simulink model "Speed_c_code_Testing_Pract"  (R2022a)
settings: Solver=VariableStepAuto  StartTime=0.0  StopTime=10  RelTol=1e-3
undefined symbols (not defined in the file or in its folder): d, F_0, F_0k, g, m, M, P_0, P_0k, PD_s, PI_s, Ts, V_0, V_0k
settings Model: Creator=DELL  LastModifiedBy=DELL

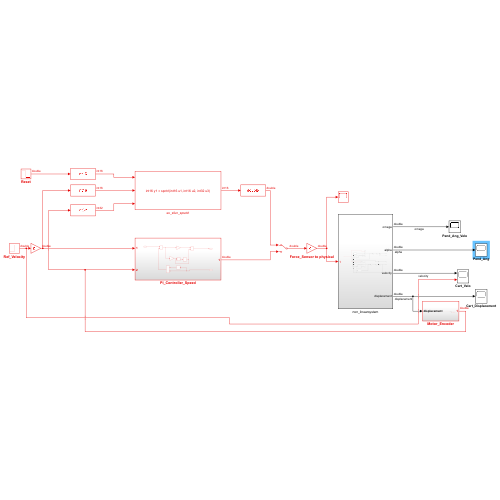
[thumbnail: Simulink's stored preview of the top-level diagram]
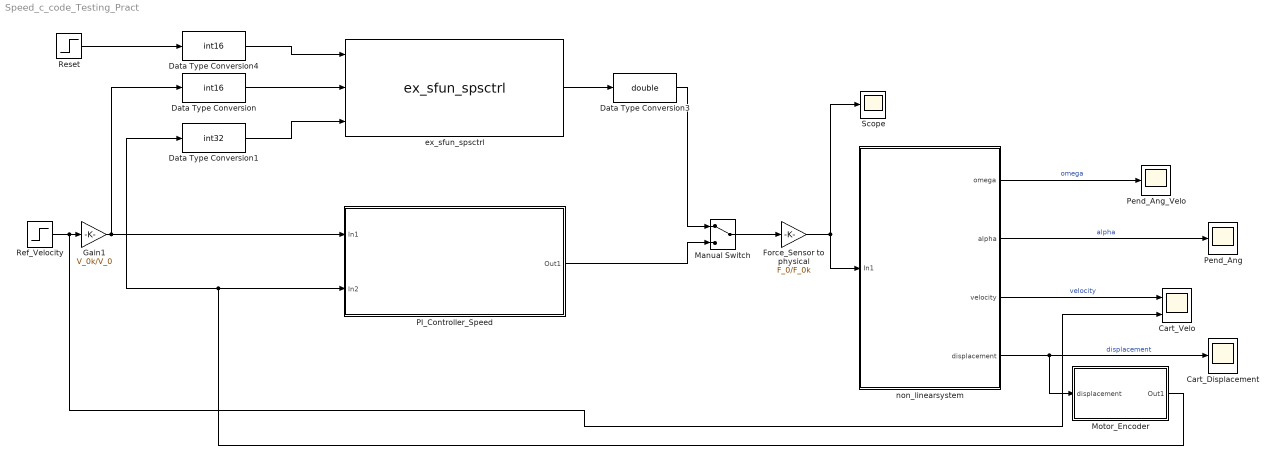
== system Speed_c_code_Testing_Pract ==
  Cart_Displacement : Scope
  Cart_Velo : Scope  NumInputPorts=2
  Data Type Conversion : DataTypeConversion  OutDataTypeStr=int16  SaturateOnIntegerOverflow=off  RndMeth=Floor
  Data Type Conversion1 : DataTypeConversion  OutDataTypeStr=int32  SaturateOnIntegerOverflow=off  RndMeth=Floor
  Data Type Conversion3 : DataTypeConversion  OutDataTypeStr=double  SaturateOnIntegerOverflow=off  RndMeth=Floor
  Data Type Conversion4 : DataTypeConversion  OutDataTypeStr=int16  SaturateOnIntegerOverflow=off  RndMeth=Floor
  Force_Sensor to physical : Gain  Gain=F_0/F_0k
  Gain1 : Gain  Gain=V_0k/V_0
  Manual Switch : ManualSwitch
  Motor_Encoder : Subsystem
  PI_Controller_Speed : Subsystem
  Pend_Ang : Scope
  Pend_Ang_Velo : Scope
  Ref_Velocity : Step  SampleTime=Ts
  Reset : Step  Time=2*Ts  Before=1  After=0  SampleTime=Ts
  Scope : Scope
  ex_sfun_spsctrl : S-Function  FunctionName=ex_sfun_spsctrl  SFunctionDeploymentMode=off  EnableBusSupport=off  mask(Legacy Function){SFunctionSpec=int16 y1 = spctrl(int16 u1, int16 u2, int32 u3), ShowSpec=on}
      mask prompts: ShowSpec "Display function specification"
      mask help:
      | This block allows you to call the legacy functions specified by the following Legacy Code Tool definition:
      | def.SFunctionName = 'ex_sfun_spsctrl';
      | def.OutputFcnSpec = 'int16 y1 = spctrl(int16 u1, int16 u2, int32 u3)';
      | def.HeaderFiles = {'xil_types.h', 'Fixedpt_Speed_Control.h'};
      mask Help: <p>This block was generated automatically by the Legacy Code Tool. For detailed help on this tool, call<a href="matlab:legacy_code('help')"> legacy_code('help')</a>.</p>
      mask Callback ShowSpec:
      | if strcmp(get_param(gcbh, 'ShowSpec'), 'on')
      |   set_param(gcbh, 'MaskDisplay', sprintf('fprintf(''%s'');', get_param(gcbh, 'SFunctionSpec')));
      | else
      |   set_param(gcbh, 'MaskDisplay', sprintf('fprintf(''%s'');', get_param(gcbh, 'FunctionName')));
      | end
      mask Display: fprintf('int16 y1 = spctrl(int16 u1, int16 u2, int32 u3)');
  non_linearsystem : Subsystem
  wires:
  non_linearsystem/1(omega) -> Pend_Ang_Velo/1  "omega"
  non_linearsystem/2(alpha) -> Pend_Ang/1  "alpha"
  non_linearsystem/3(velocity) -> Cart_Velo/1  "velocity"
  non_linearsystem/4(displacement) -> Motor_Encoder/1(displacement), Cart_Displacement/1  "displacement"
  Data Type Conversion1/1 -> ex_sfun_spsctrl/3
  ex_sfun_spsctrl/1 -> Data Type Conversion3/1
  Data Type Conversion3/1 -> Manual Switch/1
  Manual Switch/1 -> Force_Sensor to physical/1
  Data Type Conversion/1 -> ex_sfun_spsctrl/2
  Reset/1 -> Data Type Conversion4/1
  Data Type Conversion4/1 -> ex_sfun_spsctrl/1
  Force_Sensor to physical/1 -> non_linearsystem/1(In1), Scope/1
  PI_Controller_Speed/1(Out1) -> Manual Switch/2
  Ref_Velocity/1 -> Cart_Velo/2, Gain1/1
  Motor_Encoder/1(Out1) -> Data Type Conversion1/1, PI_Controller_Speed/2(In2)
  Gain1/1 -> Data Type Conversion/1, PI_Controller_Speed/1(In1)

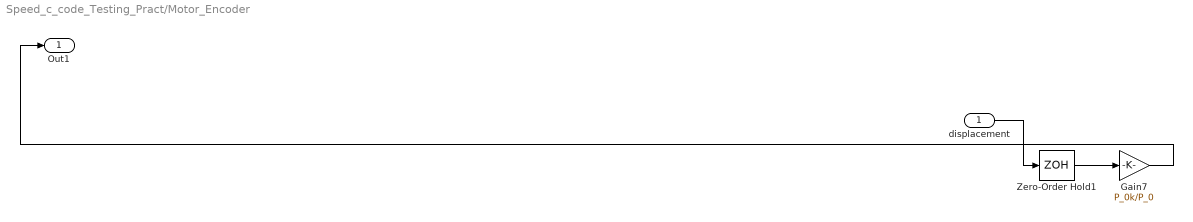
== system Speed_c_code_Testing_Pract/Motor_Encoder ==
  displacement : Inport
  Gain7 : Gain  Gain=P_0k/P_0
  Zero-Order Hold1 : ZeroOrderHold  SampleTime=Ts
  Out1 : Outport
  wires:
  Zero-Order Hold1/1 -> Gain7/1
  Gain7/1 -> Out1/1
  displacement/1 -> Zero-Order Hold1/1

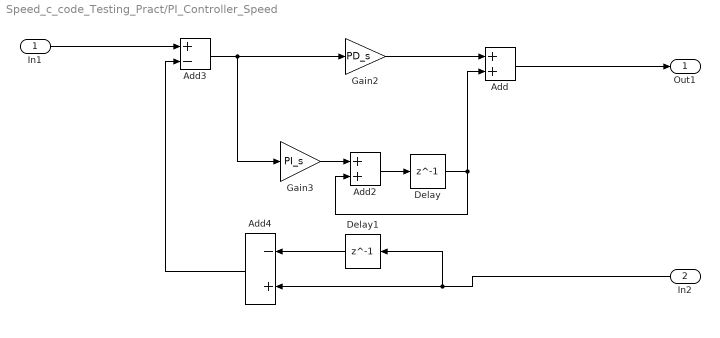
== system Speed_c_code_Testing_Pract/PI_Controller_Speed ==
  In1 : Inport
  In2 : Inport  Port=2
  Add : Sum
  Add2 : Sum
  Add3 : Sum  Inputs=+-
  Add4 : Sum  Inputs=-+
  Delay : Delay  DelayLength=1  SampleTime=Ts
  Delay1 : Delay  DelayLength=1  InitialCondition=0  SampleTime=Ts
  Gain2 : Gain  Gain=PD_s
  Gain3 : Gain  Gain=PI_s
  Out1 : Outport
  wires:
  Add/1 -> Out1/1
  Add3/1 -> Gain3/1, Gain2/1
  Gain2/1 -> Add/1
  Delay1/1 -> Add4/1
  Delay/1 -> Add/2, Add2/2
  In2/1 -> Add4/2, Delay1/1
  Add4/1 -> Add3/2
  Gain3/1 -> Add2/1
  Add2/1 -> Delay/1
  In1/1 -> Add3/1

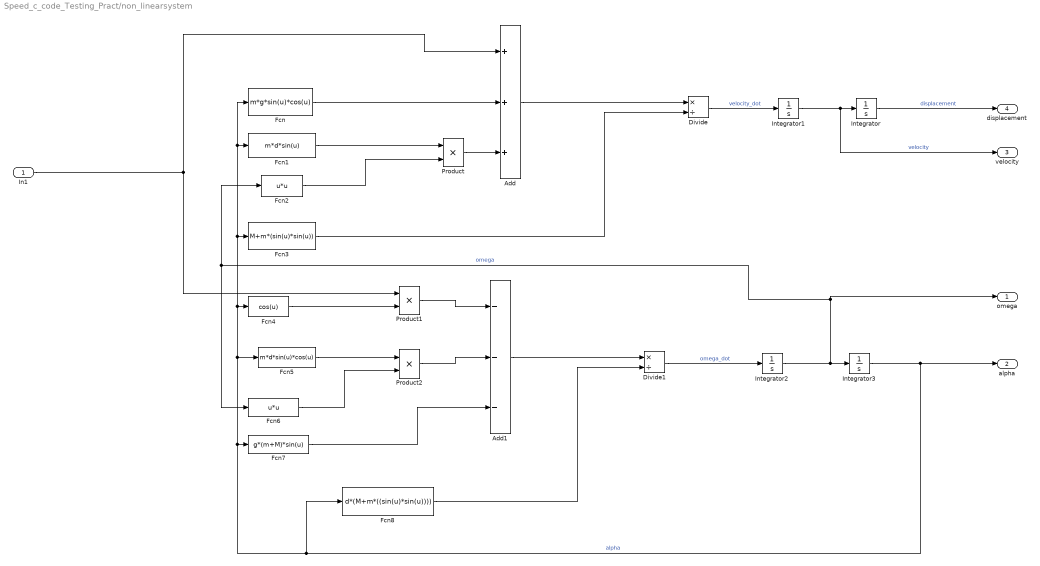
== system Speed_c_code_Testing_Pract/non_linearsystem ==
  In1 : Inport
  Add : Sum  Inputs=+++
  Add1 : Sum  Inputs=---
  Divide : Product  Inputs=*/
  Divide1 : Product  Inputs=*/
  Fcn : Fcn  Expr=m*g*sin(u)*cos(u)
  Fcn1 : Fcn  Expr=m*d*sin(u)
  Fcn2 : Fcn  Expr=u*u
  Fcn3 : Fcn  Expr=M+m*(sin(u)*sin(u))
  Fcn4 : Fcn  Expr=cos(u)
  Fcn5 : Fcn  Expr=m*d*sin(u)*cos(u)
  Fcn6 : Fcn  Expr=u*u
  Fcn7 : Fcn  Expr=g*(m+M)*sin(u)
  Fcn8 : Fcn  Expr=d*(M+m*((sin(u)*sin(u))))
  Integrator{,1..3} (4 alike) : Integrator
  Product : Product
  Product1 : Product
  Product2 : Product
  omega : Outport  VectorParamsAs1DForOutWhenUnconnected=off
  alpha : Outport  Port=2  VectorParamsAs1DForOutWhenUnconnected=off
  velocity : Outport  Port=3  VectorParamsAs1DForOutWhenUnconnected=off
  displacement : Outport  Port=4  VectorParamsAs1DForOutWhenUnconnected=off
  wires:
  Add/1 -> Divide/1
  Integrator2/1 -> Integrator3/1, omega/1, Fcn2/1, Fcn6/1  "omega"
  Fcn1/1 -> Product/1
  Integrator/1 -> displacement/1  "displacement"
  Fcn6/1 -> Product2/2
  Product/1 -> Add/3
  Fcn2/1 -> Product/2
  Fcn4/1 -> Product1/2
  Fcn/1 -> Add/2
  Integrator3/1 -> alpha/1, Fcn8/1, Fcn7/1, Fcn5/1, Fcn4/1, Fcn/1, Fcn1/1, Fcn3/1  "alpha"
  Divide/1 -> Integrator1/1  "velocity_dot"
  Fcn3/1 -> Divide/2
  Product2/1 -> Add1/2
  Add1/1 -> Divide1/1
  Fcn5/1 -> Product2/1
  Product1/1 -> Add1/1
  Fcn8/1 -> Divide1/2
  Fcn7/1 -> Add1/3
  In1/1 -> Add/1, Product1/1
  Integrator1/1 -> Integrator/1, velocity/1  "velocity"
  Divide1/1 -> Integrator2/1  "omega_dot"
